simulink model "Vehicle_Model_WIP"  (R2019b)
settings: Solver=FixedStepDiscrete  StartTime=0.0  StopTime=Simulink.t_end  FixedStep=Simulink.dt  RelTol=1e-3
undefined symbols (not defined in the file): BRK, BTRRAD, CHLR, CHRG, DCDC, DiscIntNeverNeededParam, FAN, INV, MTR, PTRAD, PUMP, Settings, TRSM, Vehicle, VHCL, WHL
libraries: simulink x8, EV_cooling x6, EV_VLD x5, EV_ePWT x5
(part 2 of 5)

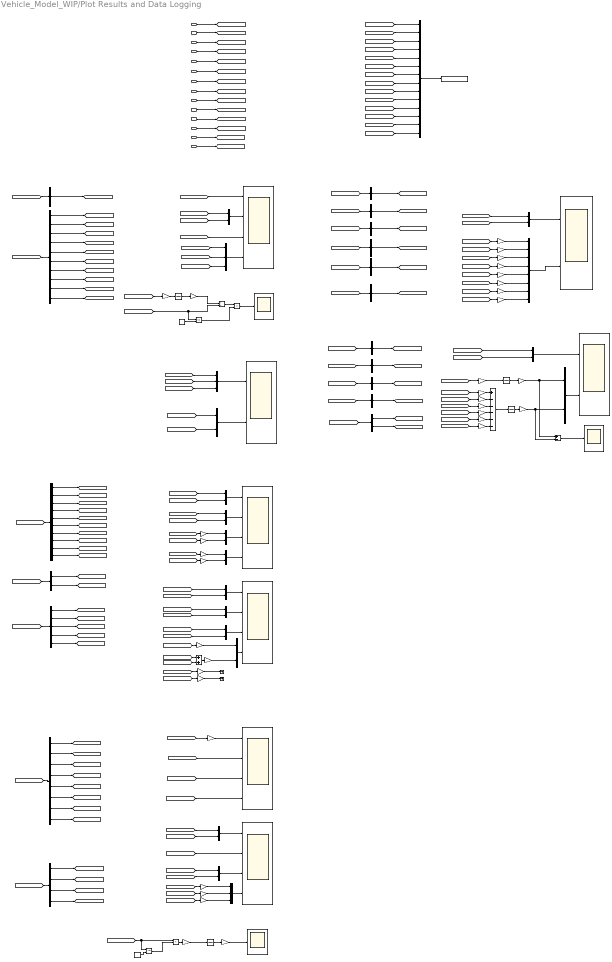
== system Vehicle_Model_WIP/Plot Results and Data Logging ==
  note: Data Logging
  note: Vehicle
  note: Motors and Cooling System
  note: Battery and Cooling system
  note: Power
  note: Energy conservation
  note: Block for visualize data and for logging to matlab workspace.
  INPT : Inport
  INIT : Inport  Port=2
  DRV : Inport  Port=3
  BTR : Inport  Port=4
  CHRG : Inport  Port=5
  DCDC : Inport  Port=6
  DC : Inport  Port=7
  INV : Inport  Port=8
  MTR : Inport  Port=9
  TRSM : Inport  Port=10
  BRK : Inport  Port=11
  CS : Inport  Port=12
  VLD : Inport  Port=13
  VCU : Inport  Port=14
  Add : Sum
  Add2 : Sum  Inputs=+-
  Add6 : Sum  Inputs=+-----
  Bus Creator : BusCreator  Inputs=14
  Bus Selector : BusSelector  OutputSignals=INPT_vReq_kph
  Bus Selector1 : BusSelector  OutputSignals=VLD_lActVhcl_km,VLD_vActVhcl_kph,VLD_aActVhcl_mps2,VLD_FTot_N,VLD_FWhl_N,VLD_FRst_N,VLD_vWhlFr_kph,VLD_vWhlRr_kph,VLD_rSlipFrt,VLD_rSlipRr
  Bus Selector10 : BusSelector  OutputSignals=INV_PwrOut_W
  Bus Selector11 : BusSelector  OutputSignals=VLD_PWhl_W
  Bus Selector12 : BusSelector  OutputSignals=DCDC_PwrAux_W
  Bus Selector13 : BusSelector  OutputSignals=INV_PwrLosses_W
  Bus Selector14 : BusSelector  OutputSignals=VLD_PWhlMtr_W,VLD_PTSlipLoss_W
  Bus Selector15 : BusSelector  OutputSignals=BRK_Pwr_W
  Bus Selector16 : BusSelector  OutputSignals=MTR_PThrmTot_W
  Bus Selector17 : BusSelector  OutputSignals=TRSM_PwrLosses_W
  Bus Selector2 : BusSelector  OutputSignals=BTR_iPackEst_A,BTR_VPackEst_V,BTR_PPackEst_W,BTR_SocPack_Ptc,BTR_TMxCell_degC,BTR_TMxBsbr_C,BTR_TWtrOut_degC,BTR_HR_pack_W
  Bus Selector20 : BusSelector  OutputSignals=DC_PBtrReq_W
  Bus Selector4 : BusSelector  OutputSignals=CS_BTR_TWtrOut_degC,CS_RAD_HeatRej_W,CS_CHLR_HeatRej_W,CS_BTR_dV_lpm
  Bus Selector5 : BusSelector  OutputSignals=MTR_rEffFrt,MTR_rEffRr,MTR_TFrtMtr_Nm,MTR_TRrMtr_Nm,MTR_PElecFrt_W,MTR_PElecRr_W,MTR_PThrmFrt_W,MTR_PThrmRr_W,MTR_TEstFrt_degC,MTR_TEstRr_degC
  Bus Selector6 : BusSelector  OutputSignals=TRSM_nMtrFrt_rpm,TRSM_nMtrRr_rpm
  Bus Selector7 : BusSelector  OutputSignals=CS_MF_TWtrIn_degC,CS_MR_TWtrIn_degC,CS_RAD_HeatRej_W,rEDU_PUMPdm,fEDU_PUMPdm
  Bus Selector8 : BusSelector  OutputSignals=MTR_PMechTot_W
  Bus Selector9 : BusSelector  OutputSignals=TRSM_PwrWhl_W
  Constant : Constant  Value=0.1
  Constant1 : Constant  Value=0
  Discrete-Time Integrator{1..4} (4 alike) : DiscreteIntegrator  SampleTime=-1  ICPrevOutput=DiscIntNeverNeededParam  ICPrevScaledInput=DiscIntNeverNeededParam
  Divide : Product  Inputs=*/
  Divide1 : Product
  Divide2 : Product  Inputs=**
  Gain{,1..4,7..14,17..21,23..24,26..30,33} (26 alike) : Gain  Gain=1e-3
  Gain15 : Gain  Gain=-1e-3
  Gain{16,25,31..32} (4 alike) : Gain  Gain=1/3600
  Gain5 : Gain  Gain=100
  Gain6 : Gain  Gain=100
  Mux{,1..2,4..7,9..12,14,16,20..21} (15 alike) : Mux  Inputs=2
  Mux13 : Mux  Inputs=8
  Mux15 : Mux  Inputs=3
  Mux3 : Mux  Inputs=3
  Mux8 : Mux  Inputs=3
  Relational Operator : RelationalOperator  OutDataTypeStr=boolean  RndMeth=Simplest
  Relational Operator1 : RelationalOperator  Operator=<=  OutDataTypeStr=boolean  RndMeth=Simplest
  Scope{,1..4} (5 alike) : Scope  NumInputPorts=4
  Scope13 : Scope  NumInputPorts=2
  Scope5 : Scope  NumInputPorts=2
  Scope6 : Scope
  Scope7 : Scope
  Scope8 : Scope
  Scope9 : Scope  NumInputPorts=2
  Terminator : Terminator
  Terminator1 : Terminator
  To Workspace : ToWorkspace  VariableName=Sim_Results  SaveFormat=Timeseries  SampleTime=-1
      settings: Save2DSignal=2-D array (concatenate along first dimension)
  wires:
  Mux/1 -> Scope/2
  [INPT_vReq_kph] -> Mux/1  "DRV_vReq_kph"
  [VLD_vActVhcl_kph] -> Mux/2  "VLD_vActVhcl_kph"
  TRSM/1 -> [TRSM]
  INV/1 -> [INV]
  INPT/1 -> [INPT]
  MTR/1 -> [MTR]
  BRK/1 -> [BRK]
  DRV/1 -> [DRV]
  BTR/1 -> [BTR]
  VLD/1 -> [VLD]
  [INPT] -> Bus Creator/1  "INPT"
  [DRV] -> Bus Creator/3  "DVR"
  [BTR] -> Bus Creator/4  "BTR"
  Bus Creator/1 -> To Workspace/1
  [INPT] -> Bus Selector/1
  Bus Selector/1 -> [INPT_vReq_kph]  "<INPT_vReq_kph>"
  [VLD] -> Bus Selector1/1
  Bus Selector1/2 -> [VLD_vActVhcl_kph]  "<VLD_vActVhcl_kph>"
  Bus Selector1/1 -> [VLD_lActVhcl_km]  "<VLD_lActVhcl_km>"
  [VLD_lActVhcl_km] -> Scope/1  "VLD_lActVhcl_km"
  INIT/1 -> [INIT]
  [INIT] -> Bus Creator/2  "INIT"
  [BTR] -> Bus Selector2/1
  Bus Selector2/1 -> [BTR_iPackEst_A]  "<BTR_iPackEst_A>"
  Bus Selector2/2 -> [BTR_VPackEst_V]  "<BTR_VPackEst_V>"
  Bus Selector2/3 -> [BTR_PPackEst_W]  "<BTR_PPackEst_W>"
  Bus Selector2/4 -> [BTR_SocPack_Ptc]  "<BTR_SocPack_Ptc>"
  Bus Selector2/5 -> [BTR_TMxCell_degC]  "<BTR_TMxCell_degC>"
  Bus Selector2/6 -> [BTR_TMxBsbr_C]  "<BTR_TMxBsbr_C>"
  Bus Selector2/7 -> [BTR_TWtrOut_degC]  "<BTR_TWtrOut_degC>"
  [BTR_PPackEst_W] -> Gain/1
  [BTR_VPackEst_V] -> Scope1/2
  [BTR_iPackEst_A] -> Scope1/3
  [BTR_SocPack_Ptc] -> Scope1/4
  Gain/1 -> Scope1/1
  Mux1/1 -> Scope2/1
  [CS] -> Bus Selector4/1
  Bus Selector4/1 -> [BCS_TWtrOut_degC]  "<CS_BTR_TWtrOut_degC>"
  Bus Selector4/2 -> [CS_RAD_HeatRej_W]  "<CS_RAD_HeatRej_W>"
  Bus Selector4/3 -> [BCS_PHeatRejChlr_W]  "<CS_CHLR_HeatRej_W>"
  [BTR_TMxBsbr_C] -> Mux1/2
  [BTR_TMxCell_degC] -> Mux1/1
  [BCS_dV_lpm] -> Scope2/2
  Mux2/1 -> Scope2/3
  [BTR_TWtrOut_degC] -> Mux2/2
  [BCS_TWtrOut_degC] -> Mux2/1
  Mux3/1 -> Scope2/4
  [CS_RAD_HeatRej_W] -> Gain1/1
  [BCS_PHeatRejChlr_W] -> Gain2/1
  Gain1/1 -> Mux3/1  "<CS_RAD_HeatRej_W>"
  Gain2/1 -> Mux3/2  "<BCS_PHeatRejChlr_kW>"
  [MTR] -> Bus Selector5/1
  Bus Selector5/1 -> [MTR_rEffFrt]  "<MTR_rEffFrt>"
  Bus Selector5/2 -> [MTR_rEffRr]  "<MTR_rEffRr>"
  Bus Selector5/3 -> [MTR_TFrtMtr_Nm]  "<MTR_TFrtMtr_Nm>"
  Bus Selector5/4 -> [MTR_TRrMtr_Nm]  "<MTR_TRrMtr_Nm>"
  Bus Selector5/5 -> [MTR_PElecFrt_W]  "<MTR_PElecFrt_W>"
  Bus Selector5/6 -> [MTR_PElecRr_W]  "<MTR_PElecRr_W>"
  [TRSM] -> Bus Selector6/1
  Bus Selector6/1 -> [TRSM_nMtrFrt_rpm]  "<TRSM_nMtrFrt_rpm>"
  Bus Selector6/2 -> [TRSM_nMtrRr_rpm]  "<TRSM_nMtrRr_rpm>"
  Mux4/1 -> Scope3/1
  [MTR_TRrMtr_Nm] -> Mux4/2
  [MTR_TFrtMtr_Nm] -> Mux4/1
  Mux7/1 -> Scope3/4
  Mux6/1 -> Scope3/3
  Mux5/1 -> Scope3/2
  [TRSM_nMtrFrt_rpm] -> Mux5/1
  [TRSM_nMtrRr_rpm] -> Mux5/2
  [MTR_PElecFrt_W] -> Gain3/1
  [MTR_PElecRr_W] -> Gain4/1
  [MTR_rEffFrt] -> Gain5/1
  [MTR_rEffRr] -> Gain6/1
  Gain3/1 -> Mux6/1  "<MTR_PElecFrt_kW>"
  Gain4/1 -> Mux6/2  "<MTR_PElecRr_kW>"
  Gain5/1 -> Mux7/1  "<MTR_EffFrt_pct>"
  Gain6/1 -> Mux7/2  "<MTR_EffRr_pct>"
  Bus Selector1/3 -> [VLD_aActVhcl_mps2]  "<VLD_aActVhcl_mps2>"
  [VLD_aActVhcl_mps2] -> Scope/3
  Mux8/1 -> Scope/4
  Bus Selector5/9 -> [MTR_TEstFrt_degC]  "<MTR_TEstFrt_degC>"
  Bus Selector5/10 -> [MTR_TEstRr_degC]  "<MTR_TEstRr_degC>"
  [CS] -> Bus Selector7/1
  Mux9/1 -> Scope4/1
  [MTR_TEstFrt_degC] -> Mux9/1
  [MTR_TEstRr_degC] -> Mux9/2
  Mux12/1 -> Scope4/2
  Mux10/1 -> Scope4/3
  [CS_MF_TWtrIn_degC] -> Mux10/1
  [CS_MR_TWtrIn_degC] -> Mux10/2
  [CS_RAD_HeatRej_W2] -> Gain7/1
  Gain7/1 -> Mux11/1  "CS_RAD_HeatRej_W"
  Bus Selector5/8 -> [MTR_PThrmRr_W]  "<MTR_PThrmRr_W>"
  Bus Selector5/7 -> [MTR_PThrmFrt_W]  "<MTR_PThrmFrt_W>"
  [MTR_PThrmRr_W] -> Add/2
  [MTR_PThrmFrt_W] -> Add/1
  Mux11/1 -> Scope4/4
  Gain8/1 -> Mux11/2  "MTR_PThrmTot_kW"
  Add/1 -> Gain8/1
  Bus Selector1/4 -> [VLD_FTot_N]  "<VLD_FTot_N>"
  Bus Selector1/6 -> [VLD_FRst_N]  "<VLD_FRst_N>"
  Bus Selector1/5 -> [VLD_FWhl_N]  "<VLD_FWhl_N>"
  [VLD_FRst_N] -> Mux8/3  "FRst_N"
  [VLD_FWhl_N] -> Mux8/2  "FWhl_N"
  [INV] -> Bus Selector10/1
  VCU/1 -> [VCU]
  Bus Selector10/1 -> [INV_PwrOut_W]  "<INV_PwrOut_W>"
  [MTR] -> Bus Selector8/1
  [TRSM] -> Bus Selector9/1
  [VLD] -> Bus Selector11/1
  Bus Selector8/1 -> [MTR_PMechTot_W]  "<MTR_PMechTot_W>"
  Bus Selector9/1 -> [TRSM_PwrWhl_W]  "<TRSM_PwrWhl_W>"
  Bus Selector11/1 -> [VLD_PWhl_W]  "<VLD_PWhl_W>"
  Mux13/1 -> Scope5/2
  [DC_PBtrReq_W] -> Gain9/1
  [INV_PwrOut_W] -> Gain10/1
  [VLD_PWhl_W] -> Gain13/1
  [TRSM_PwrWhl_W] -> Gain12/1
  [MTR_PMechTot_W] -> Gain11/1
  Gain9/1 -> Mux13/1  "<BTR_PPackEst_kW>"
  Gain10/1 -> Mux13/2  "<INV_PwrOut_kW>"
  Gain11/1 -> Mux13/3  "<MTR_PMechTot_kW>"
  Gain12/1 -> Mux13/4  "<TRSM_PwrWhl_kW>"
  Gain13/1 -> Mux13/5  "<VLD_PWhl_kW>"
  [INPT_vReq_kph] -> Mux14/1  "DRV_vReq_kph"
  [VLD_vActVhcl_kph] -> Mux14/2  "VLD_vActVhcl_kph"
  Mux14/1 -> Scope5/1
  DC/1 -> [DC]
  DCDC/1 -> [DCDC]
  [DCDC] -> Bus Selector12/1
  Bus Selector12/1 -> [DCDC_PwrAux_W]  "<DCDC_PwrAux_W>"
  [DCDC_PwrAux_W] -> Gain14/1
  Gain14/1 -> Mux13/6  "<DCDC_PwrAux_kW>"
  [DCDC] -> Bus Creator/6  "DCDC"
  [VCU] -> Bus Creator/14  "VCU"
  [DC] -> Bus Creator/7  "DC"
  [INV] -> Bus Creator/8  "INV"
  [MTR] -> Bus Creator/9  "MTR"
  [TRSM] -> Bus Creator/10  "TRSM"
  [BRK] -> Bus Creator/11  "BRK"
  [VLD] -> Bus Creator/12  "VLD"
  [CS] -> Bus Creator/13  "CS"
  [TRSM] -> Bus Selector17/1
  [MTR] -> Bus Selector16/1
  [INV] -> Bus Selector13/1
  Bus Selector13/1 -> [INV_PwrLosses_W]  "<INV_PwrLosses_W>"
  Bus Selector16/1 -> [MTR_PThrmTot_W]  "<MTR_PThrmTot_W>"
  Bus Selector17/1 -> [TRSM_PwrLosses_W]  "<TRSM_PwrLosses_W>"
  Bus Selector14/1 -> [VLD_PWhlMtr_W]  "<VLD_PWhlMtr_W>"
  [VLD] -> Bus Selector14/1
  [BRK] -> Bus Selector15/1
  Bus Selector15/1 -> [BRK_Pwr_W]  "<BRK_Pwr_W>"
  [BRK_Pwr_W] -> Gain23/1
  Gain23/1 -> Mux13/7  "<BRK_Pwr_kW>"
  Add2/1 -> Scope7/1
  Discrete-Time Integrator2/1 -> Gain25/1
  [BTR_PPackEst_W] -> Gain24/1
  Gain24/1 -> Discrete-Time Integrator2/1
  Gain25/1 -> Divide/1  "BTR_EnrgOut_kWh"
  [VLD_lActVhcl_km] -> Relational Operator/1, Divide/2  "VLD_lActVhcl_km"
  Divide/1 -> Divide1/1
  Divide1/1 -> Scope8/1
  Relational Operator/1 -> Divide1/2
  Constant/1 -> Relational Operator/2
  Add6/1 -> Discrete-Time Integrator4/1
  Gain32/1 -> Add2/2, Mux20/2  "BRT_PminusLoss_kWh"
  Gain31/1 -> Add2/1, Mux20/1  "VLD_PWhlMtr_kWh"
  Discrete-Time Integrator4/1 -> Gain32/1
  Gain28/1 -> Add6/5
  Gain27/1 -> Add6/4
  Gain26/1 -> Add6/3
  Gain29/1 -> Add6/1
  [TRSM_PwrLosses_W] -> Gain28/1
  [MTR_PThrmTot_W] -> Gain27/1
  [INV_PwrLosses_W] -> Gain26/1
  Discrete-Time Integrator3/1 -> Gain31/1
  Mux20/1 -> Scope13/2
  [VLD_PWhlMtr_W] -> Gain30/1
  Bus Selector20/1 -> [DC_PBtrReq_W]  "<DC_PBtrReq_W>"
  [INPT_vReq_kph] -> Mux21/1  "DRV_vReq_kph"
  [VLD_vActVhcl_kph] -> Mux21/2  "VLD_vActVhcl_kph"
  Mux21/1 -> Scope13/1
  [DCDC_PwrAux_W] -> Gain33/1
  Gain33/1 -> Add6/2
  Gain30/1 -> Discrete-Time Integrator3/1
  [DC] -> Bus Selector20/1
  [DC_PBtrReq_W] -> Gain29/1
  Gain16/1 -> Scope6/1  "BTR_ChrgEnrg_kWh"
  Gain15/1 -> Discrete-Time Integrator1/1
  [BTR_PPackEst_W] -> Relational Operator1/1, Divide2/1
  Discrete-Time Integrator1/1 -> Gain16/1
  Constant1/1 -> Relational Operator1/2
  Relational Operator1/1 -> Divide2/2
  Divide2/1 -> Gain15/1
  Bus Selector1/7 -> [VLD_vWhlFr_kph]  "<VLD_vWhlFr_kph>"
  Bus Selector1/8 -> [VLD_vWhlRr_kph]  "<VLD_vWhlRr_kph>"
  Bus Selector1/9 -> [VLD_rSlipFrt]  "<VLD_rSlipFrt>"
  Bus Selector1/10 -> [VLD_rSlipRr]  "<VLD_rSlipRr>"
  Mux15/1 -> Scope9/1
  Mux16/1 -> Scope9/2
  [VLD_rSlipRr] -> Mux16/2
  [VLD_rSlipFrt] -> Mux16/1
  [VLD_vWhlRr_kph] -> Mux15/3
  [VLD_vWhlFr_kph] -> Mux15/2
  [VLD_vActVhcl_kph] -> Mux15/1
  Bus Selector14/2 -> [VLD_PTSlipLoss_W]  "<VLD_PTSlipLoss_W>"
  [VLD_PTSlipLoss_W] -> Gain17/1
  Gain17/1 -> Add6/6
  [VLD_PTSlipLoss_W] -> Gain18/1
  Gain18/1 -> Mux13/8  "<VLD_PTSlipLoss_kW>"
  CHRG/1 -> [CHRG]
  [CHRG] -> Bus Creator/5  "CHRG"
  CS/1 -> [CS]
  Bus Selector4/4 -> [BCS_dV_lpm]  "<CS_BTR_dV_lpm>"
  [rEDU_PUMPdm] -> Mux12/1  "rEDU_PUMPdm"
  [fEDU_PUMPdm] -> Mux12/2  "fEDU_PUMPdm"
  Bus Selector7/1 -> [CS_MF_TWtrIn_degC]  "<CS_MF_TWtrIn_degC>"
  Bus Selector7/2 -> [CS_MR_TWtrIn_degC]  "<CS_MR_TWtrIn_degC>"
  Bus Selector7/3 -> [CS_RAD_HeatRej_W2]  "<CS_RAD_HeatRej_W>"
  Bus Selector7/4 -> [rEDU_PUMPdm]  "<rEDU_PUMPdm>"
  Bus Selector7/5 -> [fEDU_PUMPdm]  "<fEDU_PUMPdm>"
  Bus Selector2/8 -> [BTR_HR_pack_W]  "<BTR_HR_pack_W>"
  [BTR_HR_pack_W] -> Gain19/1
  Gain19/1 -> Mux3/3  "<BTR_HR_pack_kW>"
  [MTR_PThrmFrt_W] -> Gain20/1
  [MTR_PThrmRr_W] -> Gain21/1
  Gain21/1 -> Terminator1/1  "MTR_Rr_HR_kW"
  Gain20/1 -> Terminator/1  "MTR_Fr_HR_kW"
  [VLD_FTot_N] -> Mux8/1

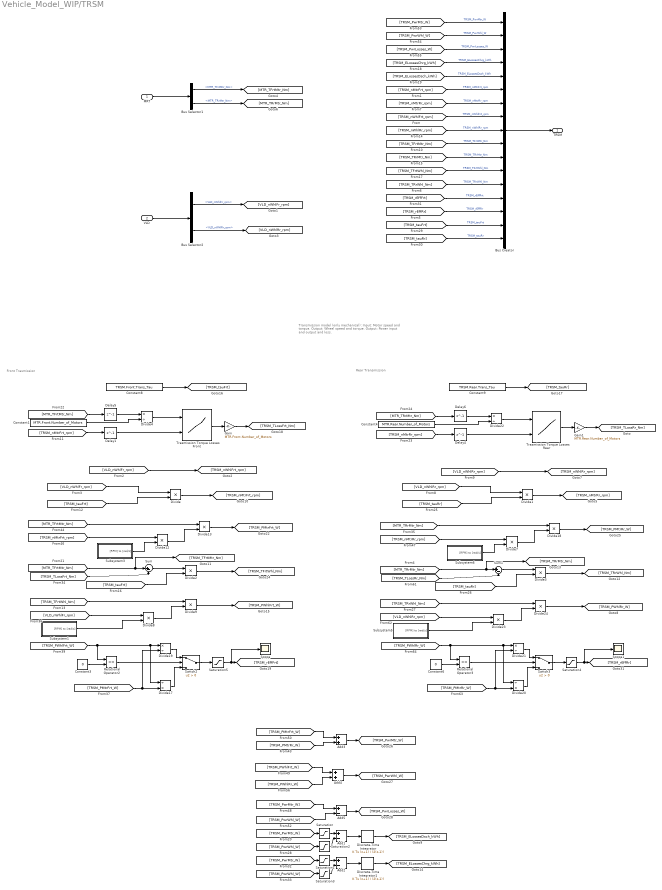
== system Vehicle_Model_WIP/TRSM ==
  note: Rear Transmission
  note: Front Trasmission
  note: Transmission model (only mechanical):
      | Input: Motor speed and torque.
      | Output: Wheel speed and torque.
      | Output: Power input and output and loss.
  MRT : Inport
  VLD : Inport  Port=2
  Add1 : Sum  Inputs=+-
  Add2 : Sum  Inputs=+-
  Add3 : Sum
  Add4 : Sum
  Add5 : Sum  Inputs=+-
  Bus Creator : BusCreator  Inputs=17
  Bus Selector1 : BusSelector  OutputSignals=MTR_TFrtMtr_Nm,MTR_TRrMtr_Nm
  Bus Selector2 : BusSelector  OutputSignals=VLD_nWhlFr_rpm,VLD_nWhlRr_rpm
  Constant1 : Constant  Value=MTR.Front.Number_of_Motors
  Constant3 : Constant  Value=0
  Constant4 : Constant  Value=MTR.Rear.Number_of_Motors
  Constant6 : Constant  Value=0
  Constant8 : Constant  Value=TRSM.Front.Trans_Tau
  Constant9 : Constant  Value=TRSM.Rear.Trans_Tau
  Delay{1,4..6} (4 alike) : Delay  DelayLength=1
  Discrete-Time Integrator : DiscreteIntegrator  IntegratorMethod=Integration: Trapezoidal  gainval=1e-3/3600  SampleTime=-1  ICPrevOutput=DiscIntNeverNeededParam  ICPrevScaledInput=DiscIntNeverNeededParam
  Discrete-Time Integrator1 : DiscreteIntegrator  IntegratorMethod=Integration: Trapezoidal  gainval=1e-3/3600  SampleTime=-1  ICPrevOutput=DiscIntNeverNeededParam  ICPrevScaledInput=DiscIntNeverNeededParam
  Divide{,1..3,7..8,12..13,18,23} (10 alike) : Product
  Divide17 : Product  Inputs=/*
  Divide{4,19,21..22} (4 alike) : Product  Inputs=*/
  Divide20 : Product  Inputs=/*
  Divide24 : Product  Inputs=**
  Divide9 : Product  Inputs=**
  Gain : Gain  Gain=MTR.Front.Number_of_Motors
  Gain1 : Gain  Gain=MTR.Rear.Number_of_Motors
  Relational Operator2 : RelationalOperator  OutDataTypeStr=boolean  RndMeth=Simplest
  Relational Operator3 : RelationalOperator  OutDataTypeStr=boolean  RndMeth=Simplest
  Saturation : Saturate  UpperLimit=inf  LowerLimit=0
  Saturation1 : Saturate  UpperLimit=0  LowerLimit=-inf
  Saturation2 : Saturate  UpperLimit=inf  LowerLimit=0
  Saturation3 : Saturate  UpperLimit=0  LowerLimit=-inf
  Saturation4 : Saturate  UpperLimit=1  LowerLimit=0
  Saturation5 : Saturate  UpperLimit=1  LowerLimit=0
  Scope : Scope
  Scope1 : Scope
  Subsystem1 : Subsystem
  Subsystem3 : Subsystem
  Subsystem5 : Subsystem
  Subsystem6 : Subsystem
  Sum : Sum  Inputs=|+-
  Sum1 : Sum  Inputs=|+-
  Switch2 : Switch  Criteria=u2 > Threshold
  Switch3 : Switch  Criteria=u2 > Threshold
  Trasmission Torque Losses Front : Lookup_n-D  BreakpointsForDimension1=TRSM.Front.bp_Torque_Nm_Mtr  BreakpointsForDimension2=TRSM.Front.bp_RPM_Mtr  Table=TRSM.Front.TLoss  ExtrapMethod=Clip  UseLastTableValue=on  RndMeth=Simplest  InputSameDT=on
  Trasmission Torque Losses Rear : Lookup_n-D  BreakpointsForDimension1=TRSM.Rear.bp_Torque_Nm_Mtr  BreakpointsForDimension2=TRSM.Rear.bp_RPM_Mtr  Table=TRSM.Rear.TLoss  ExtrapMethod=Clip  UseLastTableValue=on  RndMeth=Simplest  InputSameDT=on
  TRSM : Outport  VectorParamsAs1DForOutWhenUnconnected=off
  wires:
  Bus Creator/1 -> TRSM/1
  VLD/1 -> Bus Selector2/1
  Bus Selector2/1 -> [VLD_nWhlFr_rpm]  "<VLD_nWhlFr_rpm>"
  Bus Selector2/2 -> [VLD_nWhlRr_rpm]  "<VLD_nWhlRr_rpm>"
  MRT/1 -> Bus Selector1/1
  Bus Selector1/1 -> [MTR_TFrtMtr_Nm]  "<MTR_TFrtMtr_Nm>"
  Bus Selector1/2 -> [MTR_TRrMtr_Nm]  "<MTR_TRrMtr_Nm>"
  [VLD_nWhlFr_rpm] -> Divide/1
  [TRSM_tauFrt] -> Divide/2
  Divide/1 -> [TRSM_nMtrFrt_rpm]
  Divide1/1 -> [TRSM_nMtrRr_rpm]
  [VLD_nWhlRr_rpm] -> Divide1/1
  [TRSM_tauRr] -> Divide1/2
  [VLD_nWhlFr_rpm] -> [TRSM_nWhlFrt_rpm]
  [VLD_nWhlRr_rpm] -> [TRSM_nWhlRr_rpm]
  Constant8/1 -> [TRSM_tauFrt]
  Constant9/1 -> [TRSM_tauRr]
  Trasmission Torque Losses Front/1 -> Gain/1
  Subsystem1/1("[RPM] to [rad/s]") -> Divide8/2
  [VLD_nWhlFr_rpm] -> Divide8/1
  Divide13/1 -> [TRSM_PMtrFrt_W]
  Divide12/1 -> Divide13/2
  [MTR_TFrtMtr_Nm] -> Divide13/1
  Subsystem3/1("[RPM] to [rad/s]") -> Divide12/2
  [TRSM_PMtrRr_W] -> Add3/2
  [TRSM_PMtrFrt_W] -> Add3/1
  [TRSM_PWhlFrt_W] -> Add4/1
  [TRSM_PWhlRr_W] -> Add4/2
  Add3/1 -> [TRSM_PwrMtr_W]
  Add4/1 -> [TRSM_PwrWhl_W]
  [TRSM_PwrMtr_W] -> Add5/1
  [TRSM_PwrWhl_W] -> Add5/2
  Add5/1 -> [TRSM_PwrLosses_W]
  [TRSM_PwrWhl_W] -> Bus Creator/2  "TRSM_PwrWhl_W"
  [TRSM_PwrLosses_W] -> Bus Creator/3  "TRSM_PwrLosses_W"
  [TRSM_nMtrFrt_rpm] -> Bus Creator/6  "TRSM_nMtrFrt_rpm"
  [TRSM_nMtrRr_rpm] -> Bus Creator/7  "TRSM_nMtrRr_rpm"
  [TRSM_nWhlFrt_rpm] -> Bus Creator/8  "TRSM_nWhlFrt_rpm"
  [TRSM_nWhlRr_rpm] -> Bus Creator/9  "TRSM_nWhlRr_rpm"
  [TRSM_TFrtMtr_Nm] -> Bus Creator/10  "TRSM_TFrtMtr_Nm"
  [TRSM_TRrMtr_Nm] -> Bus Creator/11  "TRSM_TRrMtr_Nm"
  [TRSM_TFrtWhl_Nm] -> Bus Creator/12  "TRSM_TFrtWhl_Nm"
  [TRSM_TRrWhl_Nm] -> Bus Creator/13  "TRSM_TRrWhl_Nm"
  [TRSM_tauFrt] -> Bus Creator/16  "TRSM_tauFrt"
  [TRSM_tauRr] -> Bus Creator/17  "TRSM_tauRr"
  [TRSM_rEffFrt] -> Bus Creator/14  "TRSM_rEffFrt"
  [TRSM_rEffRr] -> Bus Creator/15  "TRSM_rEffRr"
  [TRSM_PwrMtr_W] -> Bus Creator/1  "TRSM_PwrMtr_W"
  Divide17/1 -> Switch2/3
  Divide19/1 -> Switch2/1
  Constant3/1 -> Relational Operator2/2
  [TRSM_PMtrFrt_W] -> Divide19/2, Divide17/2
  Relational Operator2/1 -> Switch2/2
  [TRSM_nMtrFrt_rpm] -> Delay1/1
  Constant1/1 -> Divide4/2
  [MTR_TFrtMtr_Nm] -> Delay5/1
  Delay5/1 -> Divide4/1
  [TRSM_nMtrFrt_rpm] -> Divide12/1
  [TRSM_PwrMtr_W] -> Saturation/1
  [TRSM_PwrWhl_W] -> Saturation2/1
  Saturation2/1 -> Add1/2
  Saturation/1 -> Add1/1
  Saturation1/1 -> Add2/1
  Add1/1 -> Discrete-Time Integrator/1
  Add2/1 -> Discrete-Time Integrator1/1
  [TRSM_PwrMtr_W] -> Saturation1/1
  [TRSM_PwrWhl_W] -> Saturation3/1
  Saturation3/1 -> Add2/2
  [TRSM_ELossesChrg_kWh] -> Bus Creator/4  "TRSM_ELossesChrg_kWh"
  [TRSM_ELossesDsch_kWh] -> Bus Creator/5  "TRSM_ELossesDsch_kWh"
  Discrete-Time Integrator/1 -> [TRSM_ELossesDsch_kWh]
  Discrete-Time Integrator1/1 -> [TRSM_ELossesChrg_kWh]
  Gain/1 -> [TRSM_TLossFrt_Nm]
  [TRSM_TLossFrt_Nm] -> Sum/2
  Switch2/1 -> Saturation5/1
  Divide4/1 -> Trasmission Torque Losses Front/1
  Delay1/1 -> Trasmission Torque Losses Front/2
  [TRSM_PWhlFrt_W] -> Relational Operator2/1, Divide17/1, Divide19/1
  [TRSM_PWhlRr_W] -> Divide21/1, Divide20/1, Relational Operator3/1
  Delay4/1 -> Trasmission Torque Losses Rear/2
  Divide22/1 -> Trasmission Torque Losses Rear/1
  Switch3/1 -> Saturation4/1
  Gain1/1 -> [TRSM_TLossRr_Nm]
  [TRSM_nMtrRr_rpm] -> Divide7/1
  Delay6/1 -> Divide22/1
  [MTR_TRrMtr_Nm] -> Delay6/1
  Constant4/1 -> Divide22/2
  [TRSM_nMtrRr_rpm] -> Delay4/1
  Relational Operator3/1 -> Switch3/2
  [TRSM_PMtrRr_W] -> Divide20/2, Divide21/2
  Constant6/1 -> Relational Operator3/2
  Divide21/1 -> Switch3/1
  Divide20/1 -> Switch3/3
  Subsystem6/1("[RPM] to [rad/s]") -> Divide7/2
  [MTR_TRrMtr_Nm] -> Divide18/1
  Divide7/1 -> Divide18/2
  Divide18/1 -> [TRSM_PMtrRr_W]
  Divide23/1 -> Divide24/2
  [VLD_nWhlRr_rpm] -> Divide23/1
  Subsystem5/1("[RPM] to [rad/s]") -> Divide23/2
  Trasmission Torque Losses Rear/1 -> Gain1/1
  [TRSM_TFrtWhl_Nm] -> Divide9/1
  Divide8/1 -> Divide9/2
  Saturation4/1 -> [TRSM_rEffRr], Scope1/1
  Saturation5/1 -> Scope/1, [TRSM_rEffFrt]
  [MTR_TFrtMtr_Nm] -> [TRSM_TFrtMtr_Nm], Sum/1
  Divide9/1 -> [TRSM_PWhlFrt_W]
  [TRSM_TRrWhl_Nm] -> Divide24/1
  Divide24/1 -> [TRSM_PWhlRr_W]
  Sum/1 -> Divide2/1
  [TRSM_tauFrt] -> Divide2/2
  Divide2/1 -> [TRSM_TFrtWhl_Nm]
  [MTR_TRrMtr_Nm] -> [TRSM_TRrMtr_Nm], Sum1/1
  [TRSM_TLossRr_Nm] -> Sum1/2
  Sum1/1 -> Divide3/1
  Divide3/1 -> [TRSM_TRrWhl_Nm]
  [TRSM_tauRr] -> Divide3/2

== system Vehicle_Model_WIP/VCU ==
  note: VCU architecture 2.0
  note: Front Brake command and Regenerative power
  note: Rear Brake command and Regenerative power
  note: Brakes:
      | The residual brake required (more than 0.3g --> not able to regen) is divided into a 2 to 1 ration between front and rear
  INV : Inport
  DRV : Inport  Port=2
  MTR : Inport  Port=3
  VLD : Inport  Port=4
  Bus Creator : BusCreator  Inputs=6
  Bus Selector : BusSelector  OutputSignals=VLD_vActVhcl_kph,VLD_PWhlMtr_W
  Bus Selector1 : BusSelector  OutputSignals=INV_PwrIn_W
  Bus Selector4 : BusSelector  OutputSignals=DRV_rThrottle,DRV_rBrake
  Gain : Gain  Gain=0.5
  HMI_Cruise_kph : Constant  Value=-1
  Product : Product
  Product1 : Product  Inputs=/*
  Product2 : Product  Inputs=/*
  Saturation : Saturate  UpperLimit=1  LowerLimit=0
  Setting.slip : Constant  Value=Settings.slip
  Switch : Switch
  Torque Distribution : Subsystem
  Torque Limiter : Subsystem
  Torque Request : Subsystem
  Unit Delay : UnitDelay  SampleTime=-1  HasFrameUpgradeWarning=on
  Unit Delay1 : UnitDelay  SampleTime=-1  HasFrameUpgradeWarning=on
  VLD1 : InportShadow  Port=4
  traction : Constant  Value=2
  VCU : Outport  VectorParamsAs1DForOutWhenUnconnected=off
  wires:
  Bus Selector4/1 -> [DRV_rThrottle]  "<DRV_rThrottle>"
  VLD/1 -> Bus Selector/1
  DRV/1 -> Bus Selector4/1
  Bus Selector/1 -> [VLD_vActVhcl_kph]  "<VLD_vActVhcl_kph>"
  Bus Selector4/2 -> [DRV_rBrake]  "<DRV_rBrake>"
  [VCU_rBrk] -> Gain/1
  [VCU_rBrk] -> [VCU_rBrkCmdFrt]
  [DRV_rThrottle] -> Torque Request/1(DRV_rThrottle)
  [DRV_rBrake] -> Torque Request/2(DRV_rBrake)
  HMI_Cruise_kph/1 -> Torque Request/6(HMI_Cruise_kph)
  Torque Limiter/2(TrqReqRrLim_N) -> [VCU_LimTrqRr_Nm], Torque Distribution/2(TrqReqLimRr)
  Torque Limiter/1(TrqReqFrLim_N) -> [VCU_LimTrqFr_Nm], Torque Distribution/1(TrqReqLimFr)
  VLD1/1 -> Torque Distribution/4(VLD)
  traction/1 -> Product/1
  Torque Distribution/1(TrqReqFr_Nm) -> [VCU_TInvReqFr_Nm]
  Torque Distribution/2(TrqReqRr_Nm) -> [VCU_TInvReqRr_Nm]
  Product/1 -> Torque Distribution/3(traction)
  Setting.slip/1 -> Product/2
  MTR/1 -> Torque Limiter/4(MTR)
  Torque Request/4(VCU_rBrk) -> [VCU_rBrk]
  [VCU_TInvReqFr_Nm] -> Bus Creator/1  "VCU_TInvReqFr_Nm"
  [VCU_TInvReqRr_Nm] -> Bus Creator/2  "VCU_TInvReqRr_Nm"
  [VCU_rSplitT] -> Bus Creator/3  "VCU_rSplitT"
  [VCU_rBrkCmdFrt] -> Bus Creator/4  "VCU_rBrkCmdFrt"
  Bus Creator/1 -> VCU/1
  Torque Request/1(TrqReqFr_Nm) -> Torque Limiter/1(TrqReqFr_Nm)
  Torque Request/2(TrqReqRr_Nm) -> Torque Limiter/2(TrqReqRr_Nm)
  Torque Request/3(TrqDstrRr) -> [VCU_rSplitT], Torque Limiter/3(PosTrqSplit)
  INV/1 -> Bus Selector1/1, Torque Limiter/5(INV)
  [VLD_vActVhcl_kph] -> Torque Request/3(VLD_vActVhcl_kph)
  [VCU_LimTrqFr_Nm] -> Unit Delay/1
  Unit Delay/1 -> Torque Request/4(VCU_LimTrqFr_Nm)
  [VCU_LimTrqRr_Nm] -> Unit Delay1/1
  Unit Delay1/1 -> Torque Request/5(VCU_LimTrqRr_Nm)
  [VCU_rBrkCmdRr] -> Bus Creator/5  "VCU_rBrkCmdRr"
  Gain/1 -> [VCU_rBrkCmdRr]
  Bus Selector/2 -> [VLD_PWhlMtr_W]  "<VLD_PWhlMtr_W>"
  Bus Selector1/1 -> [INV_PwrIn_W]  "<INV_PwrIn_W>"
  [VLD_PWhlMtr_W] -> Product2/1, Product1/2, Switch/2
  [INV_PwrIn_W] -> Product1/1
  [INV_PwrIn_W] -> Product2/2
  Switch/1 -> Saturation/1
  [VCU_GlobalEff] -> Bus Creator/6  "VCU_GlobalEff"
  Saturation/1 -> [VCU_GlobalEff]
  Product1/1 -> Switch/1
  Product2/1 -> Switch/3

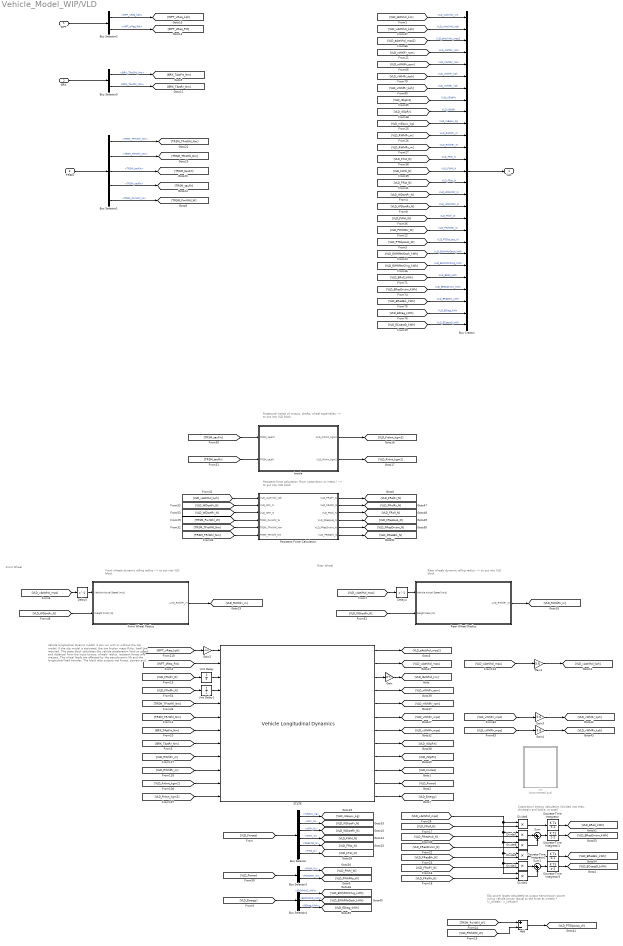
== system Vehicle_Model_WIP/VLD ==
  note: Rear Wheel
  note: Front Wheel
  note: Vehicle longitudinal dinamic model:
      | it can run with or without the slip model. If the slip model is activated, the tire friction maps f(slip, load) are required.
      | The state block calculates the vehicle acceleration (and so speed and distance) from the input torque, wheels' radius, resistant forces and masses. The wheel loads are affected by the aerodynamic lift and the longitudinal load transfer.
      | The block also outputs net forces, powers and energies useful for the post-pro of the results.
  note: Rotational inertia of motors, shafts, wheel assemblies --> to put into VLD block
  note: Resistant force calculation (from coast-down or interp.) --> to put into VLD block
  note: Front wheels dynamic rolling radius --> to put into VLD block
  note: Rear wheels dynamic rolling radius --> to put into VLD block
  note: Coast-down energy calculation (divided into tires, drivetrain and brake, or total)
  note: Slip power losses calculated as output transmission power minus vehicle power (equal to the force at wheels * (v_wheels - v_vehicle))
  INPT : Inport
  BRK : Inport  Port=2
  TRSM : Inport  Port=3
  Add : Sum  Inputs=+-
  Bus Creator : BusCreator  Inputs=27
  Bus Selector : BusSelector  OutputSignals=mequiv_kg,WFr_N,WRr_N,FWhl_N,FResTot_N,FTot_N
  Bus Selector1 : BusSelector  OutputSignals=TRSM_TFrtWhl_Nm,TRSM_TRrWhl_Nm,TRSM_tauFrt,TRSM_tauRr,TRSM_PwrWhl_W
  Bus Selector2 : BusSelector  OutputSignals=INPT_vReq_kph,INPT_sReq_Pct
  Bus Selector3 : BusSelector  OutputSignals=PWhl_W,PWhlMtr_W
  Bus Selector4 : BusSelector  OutputSignals=EWhlMtrC_kWh,EWhlMtrD_kWh,EDrag_kWh
  Bus Selector5 : BusSelector  OutputSignals=BRK_TActFrt_Nm,BRK_TActRr_Nm
  Delay4 : Delay  DelayLength=1
  Delay5 : Delay  DelayLength=1
  Discrete-Time Integrator{,1..3} (4 alike) : DiscreteIntegrator  gainval=1e-3/3600  SampleTime=-1  ICPrevOutput=DiscIntNeverNeededParam  ICPrevScaledInput=DiscIntNeverNeededParam
  Divide{1..2,6..9} (6 alike) : Product
  Front Wheel Radius : Subsystem
  Gain : Gain  Gain=1e-3
  Gain1 : Gain  Gain=3.6
  Gain2 : Gain  Gain=1/3.6
  Gain3 : Gain  Gain=3.6
  Gain4 : Gain  Gain=3.6
  Inertia : Subsystem
  Rear Wheel Radius : Subsystem
  Resistant Force Calculation : Subsystem
  STATE : EV_VLD/Vehicle Longitudinal Dynamics  slip=Settings.slip  mass_kg=VHCL.tot_mass_kg  WDFr_p=VHCL.Front_Weight_distrib_perc  l_m=VHCL.Wheelbase_mm/1000  hCOG_m=VHCL.CG_height_m  tow_mass_kg=VHCL.Towing_w_kg  h_tow=VHCL.h_tow  Tenv_degC=Settings.INIT_TEnv_degC  Fsurf_sm=VHCL.Aero_surf  Cl_Fr1=VHCL.Aero_Cl_Fr_LD  Cl_Rr1=VHCL.Aero_Cl_Rr_LD  Cd1=VHCL.Aero_Cx_LD  WRS_kmph=VHCL.Aero_WRS_kph  Cl_Fr2=VHCL.Aero_Cl_Fr_HD  Cl_Rr2=VHCL.Aero_Cl_Rr_HD  Cd2=VHCL.Aero_Cx_HD  VLoad_bp=WHL.Front.long(2:end,1)  slip_bp=WHL.Front.long(1,2:end)  frictionFr_map=VHCL.Front.mu*WHL.Front.long(2:end,2:end)  frictionRr_map=VHCL.Front.mu*WHL.Rear.long(2:end,2:end)  mu_front=VHCL.Front.mu  mu_rear=VHCL.Rear.mu
      settings: SourceProductName=EV_lib
  Sum : Sum  Inputs=|++
  Sum1 : Sum  Inputs=|++
  Unit Delay : UnitDelay  SampleTime=-1  HasFrameUpgradeWarning=on
  Unit Delay1 : UnitDelay  SampleTime=-1  HasFrameUpgradeWarning=on
  old : Subsystem  Commented=on
  VLD : Outport  VectorParamsAs1DForOutWhenUnconnected=off
  wires:
  INPT/1 -> Bus Selector2/1
  TRSM/1 -> Bus Selector1/1
  Bus Selector2/2 -> [INPT_sReq_Pct]  "<INPT_sReq_Pct>"
  Bus Selector1/1 -> [TRSM_TFrtWhl_Nm]  "<TRSM_TFrtWhl_Nm>"
  Bus Selector1/2 -> [TRSM_TRrWhl_Nm]  "<TRSM_TRrWhl_Nm>"
  BRK/1 -> Bus Selector5/1
  Bus Selector1/3 -> [TRSM_tauFrt]  "<TRSM_tauFrt>"
  Bus Selector1/4 -> [TRSM_tauRr]  "<TRSM_tauRr>"
  [TRSM_tauFrt] -> Inertia/1(TRSM_tauFrt)
  [TRSM_tauRr] -> Inertia/2(TRSM_tauRr)
  Bus Selector5/2 -> [BRK_TActRr_Nm]  "<BRK_TActRr_Nm>"
  Bus Selector5/1 -> [BRK_TActFrt_Nm]  "<BRK_TActFrt_Nm>"
  Bus Selector2/1 -> [INPT_vReq_kph]  "<INPT_vReq_kph>"
  Front Wheel Radius/1(LVD_RWhlFr_m) -> [VLD_RWhlFr_m]
  [VLD_vActVhcl_mps] -> Delay5/1
  [VLD_vActVhcl_mps] -> Delay4/1
  Rear Wheel Radius/1(LVD_RWhlRr_m) -> [VLD_RWhlRr_m]
  Inertia/1(VLD_FrtInrt_kgm2) -> [VLD_FrtInrt_kgm2]
  Inertia/2(VLD_RrInrt_kgm2) -> [VLD_RrInrt_kgm2]
  [VLD_vActVhcl_mps] -> Gain1/1
  Gain1/1 -> [VLD_vActVhcl_kph]
  Gain3/1 -> [VLD_vWhlFr_kph]
  [VLD_vWhlFr_mps] -> Gain3/1
  Gain4/1 -> [VLD_vWhlRr_kph]
  [VLD_vWhlRr_mps] -> Gain4/1
  Delay4/1 -> Rear Wheel Radius/1(Vehicle Actual Speed [m/s])
  Delay5/1 -> Front Wheel Radius/1(Vehicle Actual Speed [m/s])
  [VLD_vActVhcl_kph] -> Resistant Force Calculation/1(VLD_vActVhcl_kph)
  Bus Selector1/5 -> [TRSM_PwrWhl_W]  "<TRSM_PwrWhl_W>"
  [TRSM_PwrWhl_W] -> Add/1
  [VLD_PWhlMtr_W] -> Add/2
  Add/1 -> [VLD_PTSlipLoss_W]
  Resistant Force Calculation/1(VLD_FRolFr_N) -> [VLD_FRolFr_N]
  [VLD_WDisrtFr_N] -> Front Wheel Radius/2(Weight Front [N])
  [VLD_WDisrtRr_N] -> Rear Wheel Radius/2(Weight Rear [N])
  [VLD_WDisrtFr_N] -> Resistant Force Calculation/2(VLD_WFr_N)
  [VLD_WDisrtRr_N] -> Resistant Force Calculation/3(VLD_WRr_N)
  Resistant Force Calculation/2(VLD_FRolRr_N) -> [VLD_FRolRr_N]
  Resistant Force Calculation/3(VLD_FRoll_N) -> [VLD_FRoll_N]
  Resistant Force Calculation/4(VLD_FResHub_N) -> [VLD_FResHub_N]
  Resistant Force Calculation/5(VLD_FResDrvtrn_N) -> [VLD_FResDrvtrn_N]
  Resistant Force Calculation/6(VLD_FResBrk_N) -> [VLD_FResBrk_N]
  Discrete-Time Integrator/1 -> [VLD_ERoll_kWh]
  Discrete-Time Integrator1/1 -> [VLD_EResDrvtrn_kWh]
  Discrete-Time Integrator2/1 -> [VLD_EResBrk_kWh]
  [INPT_vReq_kph] -> Gain2/1
  [VLD_FRolFr_N] -> Unit Delay/1
  [VLD_FRolRr_N] -> Unit Delay1/1
  [INPT_sReq_Pct] -> STATE/2
  STATE/3 -> Gain/1
  STATE/1 -> [VLD_aActVhcl_mps2]
  STATE/4 -> [VLD_nWhlFr_rpm]
  STATE/5 -> [VLD_nWhlRr_rpm]
  STATE/6 -> [VLD_vWhlFr_mps]
  STATE/7 -> [VLD_vWhlRr_mps]
  STATE/8 -> [VLD_rSlipFrt]
  STATE/9 -> [VLD_rSlipRr]
  Gain/1 -> [VLD_lActVhcl_km]
  STATE/10 -> [VLD_Forces]
  STATE/11 -> [VLD_Power]
  STATE/12 -> [VLD_Energy]
  [VLD_Forces] -> Bus Selector/1
  Bus Selector/1 -> [VLD_mEquiv_kg]  "<mequiv_kg>"
  Bus Selector/2 -> [VLD_WDisrtFr_N]  "<WFr_N>"
  Bus Selector/3 -> [VLD_WDisrtRr_N]  "<WRr_N>"
  Bus Selector/4 -> [VLD_FWhl_N]  "<FWhl_N>"
  Bus Selector/5 -> [VLD_FRst_N]  "<FResTot_N>"
  Bus Selector/6 -> [VLD_FTot_N]  "<FTot_N>"
  Divide6/1 -> Discrete-Time Integrator/1
  Divide9/1 -> Discrete-Time Integrator2/1
  Divide7/1 -> Sum/1
  [VLD_FResDrvtrn_N] -> Divide8/2
  [VLD_vActVhcl_mps] -> Divide6/1, Divide2/1, Divide1/1, Divide9/1, Divide8/1, Divide7/1
  [VLD_FRoll_N] -> Divide6/2
  [VLD_FResHub_N] -> Divide7/2
  [VLD_FResBrk_N] -> Divide9/2
  Divide8/1 -> Sum/2
  Sum/1 -> Discrete-Time Integrator1/1
  [VLD_Power] -> Bus Selector3/1
  Bus Selector3/1 -> [VLD_PWhl_W]  "<PWhl_W>"
  Bus Selector3/2 -> [VLD_PWhlMtr_W]  "<PWhlMtr_W>"
  [VLD_Energy] -> Bus Selector4/1
  Bus Selector4/1 -> [VLD_EWhlMtrChrg_kWh]  "<EWhlMtrC_kWh>"
  Bus Selector4/2 -> [VLD_EWhlMtrDsch_kWh]  "<EWhlMtrD_kWh>"
  [VLD_lActVhcl_km] -> Bus Creator/1  "VLD_lActVhcl_km"
  [VLD_vActVhcl_kph] -> Bus Creator/2  "VLD_vActVhcl_kph"
  [VLD_aActVhcl_mps2] -> Bus Creator/3  "VLD_aActVhcl_mps2"
  [VLD_nWhlFr_rpm] -> Bus Creator/4  "VLD_nWhlFr_rpm"
  [VLD_nWhlRr_rpm] -> Bus Creator/5  "VLD_nWhlRr_rpm"
  [VLD_vWhlFr_kph] -> Bus Creator/6  "VLD_vWhlFr_kph"
  [VLD_vWhlRr_kph] -> Bus Creator/7  "VLD_vWhlRr_kph"
  [VLD_rSlipFrt] -> Bus Creator/8  "VLD_rSlipFrt"
  [VLD_rSlipRr] -> Bus Creator/9  "VLD_rSlipRr"
  [VLD_mEquiv_kg] -> Bus Creator/10  "VLD_mEquiv_kg"
  [VLD_RWhlFr_m] -> Bus Creator/11  "VLD_RWhlFr_m"
  [VLD_RWhlRr_m] -> Bus Creator/12  "VLD_RWhlRr_m"
  [VLD_FTot_N] -> Bus Creator/13  "VLD_FTot_N"
  [VLD_FWhl_N] -> Bus Creator/14  "VLD_FWhl_N"
  [VLD_FRst_N] -> Bus Creator/15  "VLD_FRst_N"
  [VLD_WDisrtFr_N] -> Bus Creator/16  "VLD_WDisrtFr_N"
  [VLD_WDisrtRr_N] -> Bus Creator/17  "VLD_WDisrtRr_N"
  [VLD_PWhl_W] -> Bus Creator/18  "VLD_PWhl_W"
  [VLD_PWhlMtr_W] -> Bus Creator/19  "VLD_PWhlMtr_W"
  [VLD_PTSlipLoss_W] -> Bus Creator/20  "VLD_PTSlipLoss_W"
  [VLD_EWhlMtrDsch_kWh] -> Bus Creator/21  "VLD_EWhlMtrDsch_kWh"
  [VLD_EWhlMtrChrg_kWh] -> Bus Creator/22  "VLD_EWhlMtrChrg_kWh"
  [VLD_ERoll_kWh] -> Bus Creator/23  "VLD_ERoll_kWh"
  [VLD_EResDrvtrn_kWh] -> Bus Creator/24  "VLD_EResDrvtrn_kWh"
  [VLD_EResBrk_kWh] -> Bus Creator/25  "VLD_EResBrk_kWh"
  [VLD_EDrag_kWh] -> Bus Creator/26  "VLD_EDrag_kWh"
  Bus Creator/1 -> VLD/1
  [TRSM_TFrtWhl_Nm] -> STATE/5
  [TRSM_TRrWhl_Nm] -> STATE/6
  [BRK_TActFrt_Nm] -> STATE/7
  [BRK_TActRr_Nm] -> STATE/8
  [VLD_RWhlFr_m] -> STATE/9
  [VLD_RWhlRr_m] -> STATE/10
  [VLD_FrtInrt_kgm2] -> STATE/11
  [VLD_RrInrt_kgm2] -> STATE/12
  Bus Selector4/3 -> [VLD_EDrag_kWh]  "<EDrag_kWh>"
  Gain2/1 -> STATE/1
  Unit Delay/1 -> STATE/3
  Unit Delay1/1 -> STATE/4
  [VLD_FRolFr_N] -> Divide1/2
  [VLD_FRolRr_N] -> Divide2/2
  Divide1/1 -> Sum1/1
  Divide2/1 -> Sum1/2
  Sum1/1 -> Discrete-Time Integrator3/1
  Discrete-Time Integrator3/1 -> [VLD_ECoastD_kWh]
  [VLD_ECoastD_kWh] -> Bus Creator/27  "VLD_ECoastD_kWh"
  STATE/2 -> [VLD_vActVhcl_mps]
  [TRSM_PwrWhl_W] -> Resistant Force Calculation/4(TRSM_PwrWhl_W)
  [TRSM_TFrtWhl_Nm] -> Resistant Force Calculation/5(TRSM_TFrtWhl_Nm)
  [TRSM_TRrWhl_Nm] -> Resistant Force Calculation/6(TRSM_TRrWhl_Nm)

== system Vehicle_Model_WIP/old cooling ==
  note: Battery Cooling system
  note: PowerTrain Cooling system
  note: Fan and Radiator air speed
  INIT : Inport
  BTR : Inport  Port=2
  MTR : Inport  Port=3
  VCU : Inport  Port=4
  LVD : Inport  Port=5
  Battery Cooling system : Subsystem
  Fan and air for Radiators : Subsystem
  PowerTrain Cooling system : Subsystem
  BCS : Outport
  FAN : Outport  Port=2
  PTCS : Outport  Port=3
  wires:
  Fan and air for Radiators/1(FAN) -> FAN/1, Battery Cooling system/4(FAN), PowerTrain Cooling system/1(FAN)
  LVD/1 -> Fan and air for Radiators/2(VLD)
  PowerTrain Cooling system/1(PTCS) -> PTCS/1
  INIT/1 -> PowerTrain Cooling system/2(INIT), Fan and air for Radiators/1(INIT), Battery Cooling system/1(INIT)
  VCU/1 -> PowerTrain Cooling system/4(VCU), Fan and air for Radiators/3(VCU), Battery Cooling system/3(VCU)
  Battery Cooling system/1(BCS) -> BCS/1, PowerTrain Cooling system/5(BCS)
  BTR/1 -> Battery Cooling system/2(BTR)
  MTR/1 -> PowerTrain Cooling system/3(MTR)

== system Vehicle_Model_WIP/BTR/FuelCells ==
  reqPower_W : Inport
  DRV_FC_enable : Inport  Port=2
  Constant : Constant  Value=0
  From1 : From  Commented=on  GotoTag=reqPower_W
  If : If  Commented=on
  Rate Limiter : RateLimiter  RisingSlewLimit=7667  FallingSlewLimit=-23000  SampleTimeMode=inherited  InitialCondition=20000
  Rate Limiter1 : RateLimiter  Commented=on  RisingSlewLimit=7667  FallingSlewLimit=-23000  SampleTimeMode=inherited  InitialCondition=20000
  Rate Limiter2 : RateLimiter  Commented=on  RisingSlewLimit=5750*2  FallingSlewLimit=-5750*2  SampleTimeMode=inherited  InitialCondition=20000
  Rate Limiter3 : RateLimiter  Commented=on  RisingSlewLimit=5750*2  FallingSlewLimit=-5750*2  SampleTimeMode=inherited  InitialCondition=20000
  Saturation : Saturate  UpperLimit=250000*0.95  LowerLimit=20000*0.95
  Saturation1 : Saturate  Commented=on  UpperLimit=250000*0.95  LowerLimit=20000*0.95
  Scope : Scope
  Switch : Switch  Commented=on  Criteria=u2 > Threshold  Threshold=20e3
  Switch1 : Switch  Criteria=u2 > Threshold
  actPower_W : Outport
  wires:
  Rate Limiter/1 -> Saturation/1
  reqPower_W/1 -> [reqPower_W]
  Rate Limiter1/1 -> Switch/1, Switch/2
  If/1 -> Rate Limiter1/1
  From1/1 -> If/1
  Switch/1 -> Rate Limiter2/1
  Saturation1/1 -> ?
  Rate Limiter2/1 -> Saturation1/1
  DRV_FC_enable/1 -> [DRV_FC_enable]
  [reqPower_W] -> Rate Limiter/1  "FC_reqPower_W"
  Saturation/1 -> Switch1/1  "FC_actPower_W"
  [DRV_FC_enable] -> Switch1/2
  Constant/1 -> Switch1/3
  Switch1/1 -> actPower_W/1, Scope/1  "act_FC_Power_W"

== system Vehicle_Model_WIP/DRV/Driver Model ==
  INPT_vReq_kph : Inport
  VLD_vActVhcl_kph : Inport  Port=2
  Enable : EnablePort  StatesWhenEnabling=reset
  Constant : Constant  Value=0
  Constant1 : Constant
  Constant2 : Constant  Value=0.45
  Discrete PID Controller : simulink/Continuous/PID Controller  Controller=PI  Form=Parallel  TimeDomain=Discrete-time  SampleTime=-1  IntegratorMethod=Forward Euler  FilterMethod=Forward Euler  ControllerParametersSource=internal  P=0.75  I=0.01*0  D=0  UseFilter=on  N=100  TunerSelectOption=Transfer Function Based (PID Tuner App)  InitialConditionSource=internal  InitialConditionForIntegrator=0  InitialConditionForFilter=0  DifferentiatorICPrevScaledInput=0  ExternalReset=none  TrackingMode=off  Kt=1  LimitOutput=on  UpperSaturationLimit=1  LowerSaturationLimit=0  LinearizeAsGain=off  AntiWindupMode=none  Kb=1  POutMin=[]  POutMax=[]  IOutMin=[]  IOutMax=[]  DOutMin=[]  DOutMax=[]  NOutMin=[]  NOutMax=[]  SumOutMin=[]  SumOutMax=[]  SaturationOutMin=[]  SaturationOutMax=[]  PParamMin=[]  PParamMax=[]  IParamMin=[]  IParamMax=[]  DParamMin=[]  DParamMax=[]  NParamMin=[]  NParamMax=[]  KbParamMin=[]  KbParamMax=[]  KtParamMin=[]  KtParamMax=[]  KbOutMin=[]  KbOutMax=[]  KtOutMin=[]  KtOutMax=[]  IntegratorOutMin=[]  IntegratorOutMax=[]  FilterOutMin=[]  FilterOutMax=[]  SumI1OutMin=[]  SumI1OutMax=[]  SumI2OutMin=[]  SumI2OutMax=[]  SumI3OutMin=[]  SumI3OutMax=[]  SumI4OutMin=[]  SumI4OutMax=[]  SumDOutMin=[]  SumDOutMax=[]  DifferentiatorOutMin=[]  DifferentiatorOutMax=[]  FilterDiffOutCoefMin=[]  FilterDiffOutCoefMax=[]  ReciprocalOutMin=[]  ReciprocalOutMax=[]  SumDenOutMin=[]  SumDenOutMax=[]  SumNumOutMin=[]  SumNumOutMax=[]  DivideOutMin=[]  DivideOutMax=[]  IntegratorContinuousStateAttributes=''  IntegratorStateMustResolveToSignalObject=off  IntegratorRTWStateStorageClass=Auto  FilterContinuousStateAttributes=''  FilterStateMustResolveToSignalObject=off  FilterRTWStateStorageClass=Auto  ParallelPVariant=InternalParameters  IdealPVariant=Disabled  IVariant=InternalParameters  DVariant=Disabled  IntegratorVariant=Discrete  SatVariant=Enabled  AWVariant=Passthrough  PCopyVariant=Disabled  TRVariant=Disabled  FdbkBlocksVariant=Forward  IdealPFdbkVariant=Disabled  SatFdbkVariant=Disabled  DerivativeFilterVariant=Disabled  NVariant=Disabled  NCopyVariant=Disabled_SignalSpec  FilterICVariant=Disabled  IntegratorICVariant=InternalICs  ExternalResetVariant=Disabled  TRSumVariant=Passthrough  SumFdbkVariant=Disabled  SumVariant=Sum_PI
  Divide2 : Product
  Gain2 : Gain  Gain=1/3.6
  Gain3 : Gain  Gain=1/3.6
  Lookup Table1 : Lookup  InputValues=[-2 -1 0 1]  Table=[-1 -1 0 0]
  Scope : Scope
  Scope1 : Scope  NumInputPorts=2
  Sum3 : Sum  Inputs=+-
  Switch : Switch  Criteria=u2 > Threshold  Threshold=1
  DRV_rThrottle : Outport  OutputWhenDisabled=reset  InitialOutput=0  VectorParamsAs1DForOutWhenUnconnected=off
  DRV_rBrake : Outport  Port=2  OutputWhenDisabled=reset  InitialOutput=0  VectorParamsAs1DForOutWhenUnconnected=off
  DRV_FC_enable : Outport  Port=3  OutputWhenDisabled=reset  InitialOutput=0  VectorParamsAs1DForOutWhenUnconnected=off
  wires:
  [INPT_vReq_kph] -> Gain2/1
  [VLD_vActVhcl_kph] -> Gain3/1
  VLD_vActVhcl_kph/1 -> [VLD_vActVhcl_kph]
  [DRV_rThrottle] -> DRV_rThrottle/1
  INPT_vReq_kph/1 -> [INPT_vReq_kph]
  Sum3/1 -> Discrete PID Controller/1, Divide2/2
  Discrete PID Controller/1 -> Scope/1, [DRV_rThrottle]  "DRV_rThrottle"
  Lookup Table1/1 -> Scope1/2, [DRV_rBrake]
  [DRV_rBrake] -> DRV_rBrake/1
  Gain2/1 -> Sum3/1
  Gain3/1 -> Sum3/2
  Constant2/1 -> Divide2/1
  Divide2/1 -> Scope1/1, Lookup Table1/1
  Constant/1 -> Switch/3
  [VLD_vActVhcl_kph] -> Switch/2
  Constant1/1 -> Switch/1
  Switch/1 -> [FC_enable]  "FC_enable"
  [FC_enable] -> DRV_FC_enable/1

== system Vehicle_Model_WIP/INV/Inverter Controller Current ==
  VCU_TInvReqFr_Nm : Inport
  VCU_TInvReqRr_Nm : Inport  Port=2
  INV_TMtrReqFr : Outport  VectorParamsAs1DForOutWhenUnconnected=off
  INV_TMtrReqRr : Outport  Port=2  VectorParamsAs1DForOutWhenUnconnected=off
  wires:
  VCU_TInvReqFr_Nm/1 -> [VCU_TInvReqFr_Nm]
  VCU_TInvReqRr_Nm/1 -> [VCU_TInvReqRr_Nm]
  [INV_TMtrReqRr] -> INV_TMtrReqRr/1
  [INV_TMtrReqFr] -> INV_TMtrReqFr/1
  [VCU_TInvReqRr_Nm] -> [INV_TMtrReqRr]
  [VCU_TInvReqFr_Nm] -> [INV_TMtrReqFr]

== system Vehicle_Model_WIP/TRSM/Subsystem1 ==
  Constant1 : Constant  Value=60
  Constant2 : Constant  Value=pi()
  Constant3 : Constant  Value=2
  Divide1 : Product  Inputs=*/
  Divide4 : Product
  "[RPM] to [rad/s]" : Outport  VectorParamsAs1DForOutWhenUnconnected=off
  wires:
  Constant1/1 -> Divide1/2
  Divide4/1 -> Divide1/1
  Constant2/1 -> Divide4/2
  Divide1/1 -> "[RPM] to [rad/s]"/1
  Constant3/1 -> Divide4/1

== system Vehicle_Model_WIP/TRSM/Subsystem3 ==
  Constant1 : Constant  Value=60
  Constant2 : Constant  Value=pi()
  Constant3 : Constant  Value=2
  Divide1 : Product  Inputs=*/
  Divide4 : Product
  "[RPM] to [rad/s]" : Outport  VectorParamsAs1DForOutWhenUnconnected=off
  wires:
  Constant3/1 -> Divide4/1
  Divide1/1 -> "[RPM] to [rad/s]"/1
  Constant2/1 -> Divide4/2
  Divide4/1 -> Divide1/1
  Constant1/1 -> Divide1/2

== system Vehicle_Model_WIP/TRSM/Subsystem5 ==
  Constant1 : Constant  Value=60
  Constant2 : Constant  Value=pi()
  Constant3 : Constant  Value=2
  Divide1 : Product  Inputs=*/
  Divide4 : Product
  "[RPM] to [rad/s]" : Outport  VectorParamsAs1DForOutWhenUnconnected=off
  wires:
  Constant3/1 -> Divide4/1
  Divide1/1 -> "[RPM] to [rad/s]"/1
  Constant2/1 -> Divide4/2
  Divide4/1 -> Divide1/1
  Constant1/1 -> Divide1/2

== system Vehicle_Model_WIP/TRSM/Subsystem6 ==
  Constant1 : Constant  Value=60
  Constant2 : Constant  Value=pi()
  Constant3 : Constant  Value=2
  Divide1 : Product  Inputs=*/
  Divide4 : Product
  "[RPM] to [rad/s]" : Outport  VectorParamsAs1DForOutWhenUnconnected=off
  wires:
  Constant1/1 -> Divide1/2
  Divide4/1 -> Divide1/1
  Constant2/1 -> Divide4/2
  Divide1/1 -> "[RPM] to [rad/s]"/1
  Constant3/1 -> Divide4/1

== system Vehicle_Model_WIP/VCU/Torque Distribution ==
  TrqReqLimFr : Inport
  TrqReqLimRr : Inport  Port=2
  traction : Inport  Port=3
  VLD : Inport  Port=4
  Bus Selector : BusSelector  OutputSignals=VLD_WDisrtFr_N,VLD_WDisrtRr_N,VLD_RWhlFr_m,VLD_RWhlRr_m,VLD_rSlipFrt,VLD_rSlipRr
  Constant1 : Constant  Value=MTR.Front.Number_of_Motors
  Constant2 : Constant  Value=MTR.Rear.Number_of_Motors
  Product1 : Product  Inputs=**
  Product2 : Product  Inputs=**
  Terminator : Terminator
  Terminator1 : Terminator
  TractionControl : Subsystem  TreatAsAtomicUnit=on
  TrqDistr : Subsystem  TreatAsAtomicUnit=on
  sensors PREPROCESS : Subsystem  TreatAsAtomicUnit=on
  TrqReqFr_Nm : Outport
  TrqReqRr_Nm : Outport  Port=2
  wires:
  traction/1 -> [sensors_IO]
  TrqReqLimRr/1 -> [TrqReqLimRr]
  TrqReqLimFr/1 -> [TrqReqLimFr]
  [sensors_IO] -> sensors PREPROCESS/1(sensors_IO)
  [TrqReqLimFr] -> sensors PREPROCESS/2(TrqReqFr)
  [TrqReqLimRr] -> sensors PREPROCESS/3(TrqReqRr)
  TrqDistr/1(INVTrqReqFr) -> Product2/2
  TrqDistr/3(INVTrqReqRr) -> Product1/1
  VLD/1 -> Bus Selector/1
  Bus Selector/1 -> [WDistrFr]  "<VLD_WDisrtFr_N>"
  Bus Selector/2 -> [WDistrRr]  "<VLD_WDisrtRr_N>"
  sensors PREPROCESS/1(sensors) -> [sensors], TrqDistr/4(sensors)
  [WDistrFr] -> TrqDistr/3(WDistrFr)
  [WDistrRr] -> TrqDistr/5(WDistrRr)
  Bus Selector/3 -> [RWhlFr]  "<VLD_RWhlFr_m>"
  Bus Selector/4 -> [RWhlRr]  "<VLD_RWhlRr_m>"
  [RWhlRr] -> TrqDistr/6(RWheelRr)
  [RWhlFr] -> TrqDistr/2(RWheelFr)
  Constant2/1 -> Product1/2
  Constant1/1 -> Product2/1
  [sensors] -> TractionControl/2(sensors)
  TractionControl/1(TCTrqReqFr) -> [TCTrqReqFr]
  TractionControl/2(TCTrqReqRr) -> [TCTrqReqRr]
  [TCTrqReqFr] -> TrqDistr/1(TCTrqReqFr)
  [TCTrqReqRr] -> TrqDistr/7(TCTrqReqRr)
  [rSlipFr] -> TractionControl/1(slipFr)
  [rSlipRr] -> TractionControl/3(slipRr)
  TrqDistr/4(DstrTrqReqRr) -> Terminator1/1
  TrqDistr/2(DstrTrqReqFr) -> Terminator/1
  Product2/1 -> TrqReqFr_Nm/1
  Product1/1 -> TrqReqRr_Nm/1
  Bus Selector/5 -> [rSlipFr]  "<VLD_rSlipFrt>"
  Bus Selector/6 -> [rSlipRr]  "<VLD_rSlipRr>"

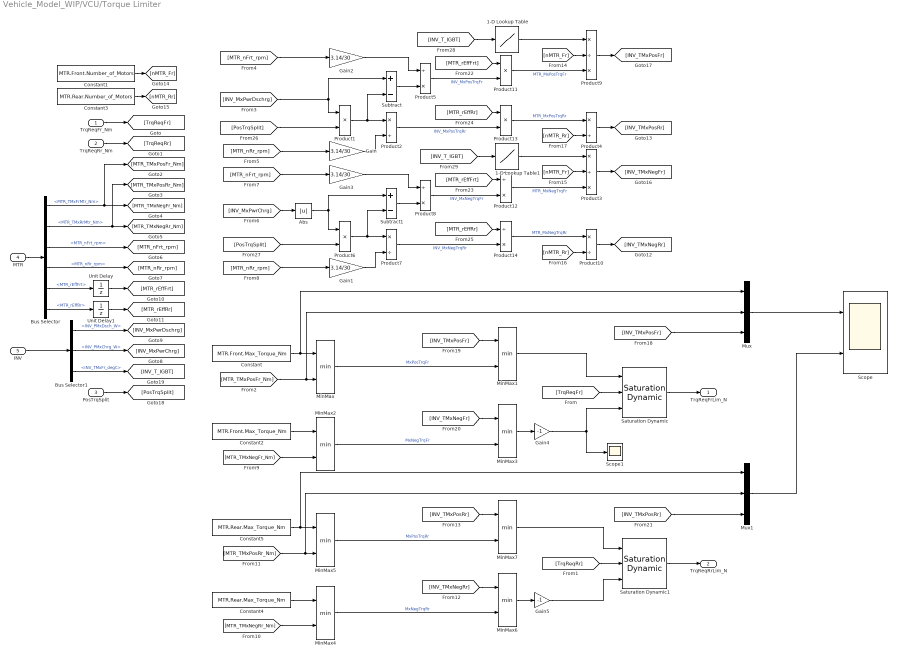
== system Vehicle_Model_WIP/VCU/Torque Limiter ==
  TrqReqFr_Nm : Inport
  TrqReqRr_Nm : Inport  Port=2
  PosTrqSplit : Inport  Port=3
  MTR : Inport  Port=4
  INV : Inport  Port=5
  1-D Lookup Table : Lookup_n-D  NumberOfTableDimensions=1  BreakpointsForDimension1=[0 150 180 190]  Table=[1 1 1 1]  InternalRulePriority=Speed  RndMeth=Simplest  InputSameDT=on
  1-D Lookup Table1 : Lookup_n-D  NumberOfTableDimensions=1  BreakpointsForDimension1=[0 150 180 190]  Table=[1 1 1 1]  InternalRulePriority=Speed  RndMeth=Simplest  InputSameDT=on
  Abs : Abs
  Bus Selector : BusSelector  OutputSignals=MTR_TMxFrMtr_Nm,MTR_TMxRrMtr_Nm,MTR_nFrt_rpm,MTR_nRr_rpm,MTR_rEffFrt,MTR_rEffRr
  Bus Selector1 : BusSelector  OutputSignals=INV_PMxDsch_W,INV_PMxChrg_W,INV_TMxFr_degC
  Constant : Constant  Value=MTR.Front.Max_Torque_Nm
  Constant1 : Constant  Value=MTR.Front.Number_of_Motors
  Constant2 : Constant  Value=MTR.Front.Max_Torque_Nm
  Constant3 : Constant  Value=MTR.Rear.Number_of_Motors
  Constant4 : Constant  Value=MTR.Rear.Max_Torque_Nm
  Constant5 : Constant  Value=MTR.Rear.Max_Torque_Nm
  Gain{,1..3} (4 alike) : Gain  Gain=3.14/30
  Gain4 : Gain  Gain=-1
  Gain5 : Gain  Gain=-1
  MinMax{,1..7} (8 alike) : MinMax  Inputs=2
  Mux : Mux  Inputs=3
  Mux1 : Mux  Inputs=3
  Product1 : Product
  Product{2,4,7,10} (4 alike) : Product  Inputs=*/
  Product11 : Product  Inputs=**
  Product{5,8,12,14} (4 alike) : Product  Inputs=/*
  Product13 : Product  Inputs=**
  Product3 : Product  Inputs=*/*
  Product6 : Product
  Product9 : Product  Inputs=*/*
  Saturation Dynamic : simulink/Discontinuities/Saturation Dynamic  OutMin=[]  OutMax=[]  OutDataTypeStr=Inherit: Same as second input  OutDataType=fixdt(1, 16)  OutScaling=2^-10  DoSatur=off
  Saturation Dynamic1 : simulink/Discontinuities/Saturation Dynamic  OutMin=[]  OutMax=[]  OutDataTypeStr=Inherit: Same as second input  OutDataType=fixdt(1, 16)  OutScaling=2^-10  DoSatur=off
  Scope : Scope  NumInputPorts=2
  Scope1 : Scope
  Subtract : Sum  Inputs=+-
  Subtract1 : Sum  Inputs=+-
  Unit Delay : UnitDelay  InitialCondition=0.8  SampleTime=-1  HasFrameUpgradeWarning=on
  Unit Delay1 : UnitDelay  InitialCondition=0.8  SampleTime=-1  HasFrameUpgradeWarning=on
  TrqReqFrLim_N : Outport
  TrqReqRrLim_N : Outport  Port=2
  wires:
  TrqReqRr_Nm/1 -> [TrqReqRr]
  TrqReqFr_Nm/1 -> [TrqReqFr]
  [MTR_TMxPosFr_Nm] -> Mux/2, MinMax/2
  Constant/1 -> Mux/1, MinMax/1
  [PosTrqSplit] -> Product1/2
  Product1/1 -> Subtract/2, Product2/1
  [MTR_nRr_rpm] -> Gain/1
  Gain/1 -> Product2/2
  Subtract/1 -> Product5/2
  [MTR_nFrt_rpm] -> Gain2/1
  [MTR_nFrt_rpm] -> Gain3/1
  Subtract1/1 -> Product8/2
  Gain1/1 -> Product7/2
  [MTR_nRr_rpm] -> Gain1/1
  Product6/1 -> Product7/1, Subtract1/2
  [PosTrqSplit] -> Product6/2
  Gain2/1 -> Product5/1
  Gain3/1 -> Product8/1
  [INV_MxPwrDschrg] -> Product1/1, Subtract/1
  Abs/1 -> Product6/1, Subtract1/1
  Product5/1 -> Product11/2  "INV_MxPosTrqFr"
  MinMax/1 -> MinMax1/2  "MxPosTrqFr"
  Constant2/1 -> MinMax2/1
  [MTR_TMxNegFr_Nm] -> MinMax2/2
  MinMax2/1 -> MinMax3/2  "MxNegTrqFr"
  MinMax3/1 -> Gain4/1
  Product8/1 -> Product12/2  "INV_MxNegTrqFr"
  [TrqReqFr] -> Saturation Dynamic/2
  Gain4/1 -> Scope1/1, Saturation Dynamic/3
  MinMax1/1 -> Saturation Dynamic/1
  Saturation Dynamic/1 -> TrqReqFrLim_N/1
  [TrqReqRr] -> Saturation Dynamic1/2
  Saturation Dynamic1/1 -> TrqReqRrLim_N/1
  Product2/1 -> Product13/2  "INV_MxPosTrqRr"
  Product7/1 -> Product14/2  "INV_MxNegTrqRr"
  [MTR_TMxNegRr_Nm] -> MinMax4/2
  Constant4/1 -> MinMax4/1
  Constant5/1 -> MinMax5/1, Mux1/1
  [MTR_TMxPosRr_Nm] -> MinMax5/2, Mux1/2
  MinMax4/1 -> MinMax6/2  "MxNegTrqRr"
  MinMax5/1 -> MinMax7/2  "MxPosTrqRr"
  MinMax6/1 -> Gain5/1
  Gain5/1 -> Saturation Dynamic1/3
  MinMax7/1 -> Saturation Dynamic1/1
  [INV_MxPwrChrg] -> Abs/1
  Mux/1 -> Scope/1
  Mux1/1 -> Scope/2
  MTR/1 -> Bus Selector/1
  Bus Selector/6 -> Unit Delay1/1  "<MTR_rEffRr>"
  Bus Selector/5 -> Unit Delay/1  "<MTR_rEffFrt>"
  Bus Selector/4 -> [MTR_nRr_rpm]  "<MTR_nRr_rpm>"
  Bus Selector/3 -> [MTR_nFrt_rpm]  "<MTR_nFrt_rpm>"
  Bus Selector/2 -> [MTR_TMxPosRr_Nm], [MTR_TMxNegRr_Nm]  "<MTR_TMxRrMtr_Nm>"
  Bus Selector/1 -> [MTR_TMxPosFr_Nm], [MTR_TMxNegFr_Nm]  "<MTR_TMxFrMtr_Nm>"
  Unit Delay/1 -> [MTR_rEffFrt]
  Unit Delay1/1 -> [MTR_rEffRr]
  Product10/1 -> [INV_TMxNegRr]
  [INV_TMxNegRr] -> MinMax6/1
  [INV_TMxPosRr] -> MinMax7/1
  Product4/1 -> [INV_TMxPosRr]
  [nMTR_Fr] -> Product9/2
  Constant1/1 -> [nMTR_Fr]
  Constant3/1 -> [nMTR_Rr]
  [nMTR_Rr] -> Product4/2
  [nMTR_Rr] -> Product10/2
  Product3/1 -> [INV_TMxNegFr]
  Product9/1 -> [INV_TMxPosFr]
  [INV_TMxPosFr] -> Mux/3
  [INV_TMxPosFr] -> MinMax1/1
  [INV_TMxNegFr] -> MinMax3/1
  [INV_TMxPosRr] -> Mux1/3
  Product11/1 -> Product9/3  "MTR_MxPosTrqFr"
  [MTR_rEffFrt] -> Product11/1
  [MTR_rEffFrt] -> Product12/1
  [MTR_rEffRr] -> Product13/1
  Product13/1 -> Product4/1  "MTR_MxPosTrqRr"
  [MTR_rEffRr] -> Product14/1
  Product14/1 -> Product10/1  "MTR_MxNegTrqRr"
  PosTrqSplit/1 -> [PosTrqSplit]
  INV/1 -> Bus Selector1/1
  Bus Selector1/3 -> [INV_T_IGBT]  "<INV_TMxFr_degC>"
  Bus Selector1/1 -> [INV_MxPwrDschrg]  "<INV_PMxDsch_W>"
  Bus Selector1/2 -> [INV_MxPwrChrg]  "<INV_PMxChrg_W>"
  [INV_T_IGBT] -> 1-D Lookup Table/1
  1-D Lookup Table/1 -> Product9/1
  [INV_T_IGBT] -> 1-D Lookup Table1/1
  Product12/1 -> Product3/3  "MTR_MxNegTrqFr"
  [nMTR_Fr] -> Product3/2
  1-D Lookup Table1/1 -> Product3/1
